simulink library "PczSimLib"  (R2022a)
settings: Solver=VariableStepAuto  StartTime=0.0  StopTime=10.0  RelTol=1e-3
undefined symbols (not defined in the file or in its folder): beta, PczSimLib_R2020b, Reshapers
libraries: dspswit3 x6, simulink x3
(part 2 of 2)

== matlab function PczSimLib/QArm blocks/Torque to pwm (corrected) 2022.04.28./Tau(u,x) ==
  data: params input; u input; x input; Tau output; mL input
function Tau = qarm_Tau(params,u,x,mL)
%#codegen

%    This function was generated by the Symbolic Math Toolbox version 8.7.
%    12-May-2021 15:32:53

%% in1 = u = dd(Theta), in2 = x = [ Theta ; d(Theta) ] , Tau = M(Theta) dd(Theta) + B(Theta) d(Theta) d(Theta) + C(Theta) d(Theta)^2 + G(Theta)
I1A = params(10,:);
I2A = params(11,:);
I3A = params(13,:);
I4A = params(15,:);
I2L = params(12,:);
I3L = params(14,:);
I4L = params(16,:);
payload = mL;
domega1 = u(1,:);
domega2 = u(2,:);
domega3 = u(3,:);
domega4 = u(4,:);
g = params(1,:);
l2 = params(2,:);
l3 = params(3,:);
lc2 = params(4,:);
lc3 = params(5,:);
lc4 = params(6,:);
m2 = params(7,:);
m3 = params(8,:);
m4 = params(9,:);
omega1 = x(5,:);
omega2 = x(6,:);
omega3 = x(7,:);
omega4 = x(8,:);
theta2 = x(2,:);
theta3 = x(3,:);
t2 = cos(theta2);
t3 = cos(theta3);
t4 = sin(theta2);
t5 = sin(theta3);
t6 = theta2+theta3;
t7 = l2.^2;
t8 = l3.^2;
t9 = lc3.^2;
t10 = omega1.^2;
t16 = -l3;
t17 = -lc2;
t18 = -lc4;
t11 = t2.^2;
t12 = l2.*t2;
t13 = cos(t6);
t14 = l2.*t5;
t15 = sin(t6);
t20 = m3.*t9;
t21 = payload.*t8;
t24 = l2.*lc3.*m3.*t3;
t25 = l2.*l3.*payload.*t3;
t27 = l2+t17;
t28 = l3+t18;
t19 = l3.*t14;
t22 = t13.^2;
t23 = t15.^2;
t26 = lc3.*m3.*t14;
t29 = -t12;
t30 = t14.*t16;
t31 = I4A.*omega1.*omega4.*t15;
t33 = t27.^2;
t34 = t28.^2;
t35 = I3A.*t13.*t15;
t36 = I4A.*t13.*t15;
t37 = I3L.*t13.*t15;
t38 = I4L.*t13.*t15;
t39 = lc3.*m3.*t12.*t13;
t40 = l3.*payload.*t12.*t13;
t42 = lc4+t14+t16;
t54 = t13.*t15.*t21;
t56 = t13.*t15.*t20;
t62 = m4.*t12.*t13.*t28;
t32 = -t26;
t41 = -t31;
t43 = t35.*2.0;
t44 = t36.*2.0;
t45 = t37.*2.0;
t46 = t38.*2.0;
t47 = t39.*2.0;
t48 = t40.*2.0;
t49 = t8+t30;
t50 = -t37;
t52 = -t38;
t57 = t54.*2.0;
t58 = t56.*2.0;
t59 = -t54;
t63 = -t56;
t65 = t62.*2.0;
t66 = m4.*t13.*t15.*t34;
t67 = m4.*t28.*t42;
t51 = -t45;
t53 = -t46;
t55 = payload.*t49;
t60 = -t57;
t64 = -t58;
t68 = t66.*2.0;
t69 = -t66;
t71 = -t67;
t61 = -t55;
t70 = -t68;
t72 = I3L+I4L+t20+t32+t61+t71;
mt1 = [domega1.*(I1A+I3A.*t22+I4A.*t22+I2L.*t11+I3L.*t23+I4L.*t23+t20.*t23+t21.*t23+I2A.*t4.^2+m3.*t7.*t11+m4.*t7.*t11+m2.*t11.*t33+m4.*t23.*t34+payload.*t7.*t11-lc3.*m3.*t12.*t15.*2.0-l3.*payload.*t12.*t15.*2.0-m4.*t12.*t15.*t28.*2.0)-omega1.*omega3.*(t43+t44+t47+t48+t51+t53+t60+t64+t65+t70)-I4A.*domega4.*t13-omega1.*omega2.*(t43+t44+t47+t48+t51+t53+t60+t64+t65+t70-I2A.*t2.*t4.*2.0+I2L.*t2.*t4.*2.0+m3.*t2.*t4.*t7.*2.0+m4.*t2.*t4.*t7.*2.0+m2.*t2.*t4.*t33.*2.0+payload.*t2.*t4.*t7.*2.0-l2.*lc3.*m3.*t4.*t15.*2.0-l2.*l3.*payload.*t4.*t15.*2.0-l2.*m4.*t4.*t15.*t28.*2.0)+I4A.*omega2.*omega4.*t15+I4A.*omega3.*omega4.*t15];
mt2 = [t41+domega2.*(I2L+I3L+I4L+t20+t21-t26.*2.0+m3.*t7+m2.*t33+payload.*t7-payload.*t19.*2.0+m4.*(l2+t28).^2)+domega3.*t72+t10.*(t35+t36+t39+t40+t50+t52+t59+t62+t63+t69-I2A.*t2.*t4+I2L.*t2.*t4+m3.*t2.*t4.*t7+m4.*t2.*t4.*t7+m2.*t2.*t4.*t33+payload.*t2.*t4.*t7-l2.*lc3.*m3.*t4.*t15-l2.*m4.*t4.*t15.*t28+l2.*payload.*t4.*t15.*t16)-omega3.^2.*(t24+l2.*m4.*t3.*t28+l2.*payload.*t3.*t16)-g.*(m3.*(t12-lc3.*t15)+m4.*(t12-t15.*t28)+payload.*(t12+t15.*t16)+m2.*t2.*t27)-omega2.*omega3.*(t24.*2.0+t25.*2.0)];
mt3 = [t41+g.*(lc3.*m3.*t15+l3.*payload.*t15+m4.*t15.*t28)+domega2.*t72+omega2.^2.*(t24+t25)+t10.*(t35+t36+t39+t40+t50+t52+t59+t62+t63+t69)+domega3.*(I3L+I4L+t20+t21+m4.*t34),I4A.*domega4-I4A.*domega1.*t13+I4A.*omega1.*omega2.*t15+I4A.*omega1.*omega3.*t15];
Tau = reshape([mt1,mt2,mt3],4,1);

== matlab function PczSimLib/QArm blocks/Torque to pwm (corrected) 2022.05.20./Tau(u,x) ==
  data: params input; u input; x input; Tau output; mL input
function Tau = qarm_Tau(params,u,x,mL)
%#codegen

%    This function was generated by the Symbolic Math Toolbox version 8.7.
%    12-May-2021 15:32:53

%% in1 = u = dd(Theta), in2 = x = [ Theta ; d(Theta) ] , Tau = M(Theta) dd(Theta) + B(Theta) d(Theta) d(Theta) + C(Theta) d(Theta)^2 + G(Theta)
I1A = params(10,:);
I2A = params(11,:);
I3A = params(13,:);
I4A = params(15,:);
I2L = params(12,:);
I3L = params(14,:);
I4L = params(16,:);
payload = mL;
domega1 = u(1,:);
domega2 = u(2,:);
domega3 = u(3,:);
domega4 = u(4,:);
g = params(1,:);
l2 = params(2,:);
l3 = params(3,:);
lc2 = params(4,:);
lc3 = params(5,:);
lc4 = params(6,:);
m2 = params(7,:);
m3 = params(8,:);
m4 = params(9,:);
omega1 = x(5,:);
omega2 = x(6,:);
omega3 = x(7,:);
omega4 = x(8,:);
theta2 = x(2,:);
theta3 = x(3,:);
t2 = cos(theta2);
t3 = cos(theta3);
t4 = sin(theta2);
t5 = sin(theta3);
t6 = theta2+theta3;
t7 = l2.^2;
t8 = l3.^2;
t9 = lc3.^2;
t10 = omega1.^2;
t16 = -l3;
t17 = -lc2;
t18 = -lc4;
t11 = t2.^2;
t12 = l2.*t2;
t13 = cos(t6);
t14 = l2.*t5;
t15 = sin(t6);
t20 = m3.*t9;
t21 = payload.*t8;
t24 = l2.*lc3.*m3.*t3;
t25 = l2.*l3.*payload.*t3;
t27 = l2+t17;
t28 = l3+t18;
t19 = l3.*t14;
t22 = t13.^2;
t23 = t15.^2;
t26 = lc3.*m3.*t14;
t29 = -t12;
t30 = t14.*t16;
t31 = I4A.*omega1.*omega4.*t15;
t33 = t27.^2;
t34 = t28.^2;
t35 = I3A.*t13.*t15;
t36 = I4A.*t13.*t15;
t37 = I3L.*t13.*t15;
t38 = I4L.*t13.*t15;
t39 = lc3.*m3.*t12.*t13;
t40 = l3.*payload.*t12.*t13;
t42 = lc4+t14+t16;
t54 = t13.*t15.*t21;
t56 = t13.*t15.*t20;
t62 = m4.*t12.*t13.*t28;
t32 = -t26;
t41 = -t31;
t43 = t35.*2.0;
t44 = t36.*2.0;
t45 = t37.*2.0;
t46 = t38.*2.0;
t47 = t39.*2.0;
t48 = t40.*2.0;
t49 = t8+t30;
t50 = -t37;
t52 = -t38;
t57 = t54.*2.0;
t58 = t56.*2.0;
t59 = -t54;
t63 = -t56;
t65 = t62.*2.0;
t66 = m4.*t13.*t15.*t34;
t67 = m4.*t28.*t42;
t51 = -t45;
t53 = -t46;
t55 = payload.*t49;
t60 = -t57;
t64 = -t58;
t68 = t66.*2.0;
t69 = -t66;
t71 = -t67;
t61 = -t55;
t70 = -t68;
t72 = I3L+I4L+t20+t32+t61+t71;
mt1 = [domega1.*(I1A+I3A.*t22+I4A.*t22+I2L.*t11+I3L.*t23+I4L.*t23+t20.*t23+t21.*t23+I2A.*t4.^2+m3.*t7.*t11+m4.*t7.*t11+m2.*t11.*t33+m4.*t23.*t34+payload.*t7.*t11-lc3.*m3.*t12.*t15.*2.0-l3.*payload.*t12.*t15.*2.0-m4.*t12.*t15.*t28.*2.0)-omega1.*omega3.*(t43+t44+t47+t48+t51+t53+t60+t64+t65+t70)-I4A.*domega4.*t13-omega1.*omega2.*(t43+t44+t47+t48+t51+t53+t60+t64+t65+t70-I2A.*t2.*t4.*2.0+I2L.*t2.*t4.*2.0+m3.*t2.*t4.*t7.*2.0+m4.*t2.*t4.*t7.*2.0+m2.*t2.*t4.*t33.*2.0+payload.*t2.*t4.*t7.*2.0-l2.*lc3.*m3.*t4.*t15.*2.0-l2.*l3.*payload.*t4.*t15.*2.0-l2.*m4.*t4.*t15.*t28.*2.0)+I4A.*omega2.*omega4.*t15+I4A.*omega3.*omega4.*t15];
mt2 = [t41+domega2.*(I2L+I3L+I4L+t20+t21-t26.*2.0+m3.*t7+m2.*t33+payload.*t7-payload.*t19.*2.0+m4.*(l2+t28).^2)+domega3.*t72+t10.*(t35+t36+t39+t40+t50+t52+t59+t62+t63+t69-I2A.*t2.*t4+I2L.*t2.*t4+m3.*t2.*t4.*t7+m4.*t2.*t4.*t7+m2.*t2.*t4.*t33+payload.*t2.*t4.*t7-l2.*lc3.*m3.*t4.*t15-l2.*m4.*t4.*t15.*t28+l2.*payload.*t4.*t15.*t16)-omega3.^2.*(t24+l2.*m4.*t3.*t28+l2.*payload.*t3.*t16)-g.*(m3.*(t12-lc3.*t15)+m4.*(t12-t15.*t28)+payload.*(t12+t15.*t16)+m2.*t2.*t27)-omega2.*omega3.*(t24.*2.0+t25.*2.0)];
mt3 = [t41+g.*(lc3.*m3.*t15+l3.*payload.*t15+m4.*t15.*t28)+domega2.*t72+omega2.^2.*(t24+t25)+t10.*(t35+t36+t39+t40+t50+t52+t59+t62+t63+t69)+domega3.*(I3L+I4L+t20+t21+m4.*t34),I4A.*domega4-I4A.*domega1.*t13+I4A.*omega1.*omega2.*t15+I4A.*omega1.*omega3.*t15];
Tau = reshape([mt1,mt2,mt3],4,1);

== matlab function PczSimLib/QArm blocks/Torque to pwm DEPRECATED/Tau(u,x) ==
  data: params input; u input; x input; Tau output; mL input
function Tau = qarm_Tau(params,u,x,mL)
%#codegen

%    This function was generated by the Symbolic Math Toolbox version 8.7.
%    12-May-2021 15:32:53

%% in1 = u = dd(Theta), in2 = x = [ Theta ; d(Theta) ] , Tau = M(Theta) dd(Theta) + B(Theta) d(Theta) d(Theta) + C(Theta) d(Theta)^2 + G(Theta)
I1A = params(10,:);
I2A = params(11,:);
I3A = params(13,:);
I4A = params(15,:);
I2L = params(12,:);
I3L = params(14,:);
I4L = params(16,:);
payload = mL;
domega1 = u(1,:);
domega2 = u(2,:);
domega3 = u(3,:);
domega4 = u(4,:);
g = params(1,:);
l2 = params(2,:);
l3 = params(3,:);
lc2 = params(4,:);
lc3 = params(5,:);
lc4 = params(6,:);
m2 = params(7,:);
m3 = params(8,:);
m4 = params(9,:);
omega1 = x(5,:);
omega2 = x(6,:);
omega3 = x(7,:);
omega4 = x(8,:);
theta2 = x(2,:);
theta3 = x(3,:);
t2 = cos(theta2);
t3 = cos(theta3);
t4 = sin(theta2);
t5 = sin(theta3);
t6 = theta2+theta3;
t7 = l2.^2;
t8 = l3.^2;
t9 = lc3.^2;
t10 = omega1.^2;
t16 = -l3;
t17 = -lc2;
t18 = -lc4;
t11 = t2.^2;
t12 = l2.*t2;
t13 = cos(t6);
t14 = l2.*t5;
t15 = sin(t6);
t20 = m3.*t9;
t21 = payload.*t8;
t24 = l2.*lc3.*m3.*t3;
t25 = l2.*l3.*payload.*t3;
t27 = l2+t17;
t28 = l3+t18;
t19 = l3.*t14;
t22 = t13.^2;
t23 = t15.^2;
t26 = lc3.*m3.*t14;
t29 = -t12;
t30 = t14.*t16;
t31 = I4A.*omega1.*omega4.*t15;
t33 = t27.^2;
t34 = t28.^2;
t35 = I3A.*t13.*t15;
t36 = I4A.*t13.*t15;
t37 = I3L.*t13.*t15;
t38 = I4L.*t13.*t15;
t39 = lc3.*m3.*t12.*t13;
t40 = l3.*payload.*t12.*t13;
t42 = lc4+t14+t16;
t54 = t13.*t15.*t21;
t56 = t13.*t15.*t20;
t62 = m4.*t12.*t13.*t28;
t32 = -t26;
t41 = -t31;
t43 = t35.*2.0;
t44 = t36.*2.0;
t45 = t37.*2.0;
t46 = t38.*2.0;
t47 = t39.*2.0;
t48 = t40.*2.0;
t49 = t8+t30;
t50 = -t37;
t52 = -t38;
t57 = t54.*2.0;
t58 = t56.*2.0;
t59 = -t54;
t63 = -t56;
t65 = t62.*2.0;
t66 = m4.*t13.*t15.*t34;
t67 = m4.*t28.*t42;
t51 = -t45;
t53 = -t46;
t55 = payload.*t49;
t60 = -t57;
t64 = -t58;
t68 = t66.*2.0;
t69 = -t66;
t71 = -t67;
t61 = -t55;
t70 = -t68;
t72 = I3L+I4L+t20+t32+t61+t71;
mt1 = [domega1.*(I1A+I3A.*t22+I4A.*t22+I2L.*t11+I3L.*t23+I4L.*t23+t20.*t23+t21.*t23+I2A.*t4.^2+m3.*t7.*t11+m4.*t7.*t11+m2.*t11.*t33+m4.*t23.*t34+payload.*t7.*t11-lc3.*m3.*t12.*t15.*2.0-l3.*payload.*t12.*t15.*2.0-m4.*t12.*t15.*t28.*2.0)-omega1.*omega3.*(t43+t44+t47+t48+t51+t53+t60+t64+t65+t70)-I4A.*domega4.*t13-omega1.*omega2.*(t43+t44+t47+t48+t51+t53+t60+t64+t65+t70-I2A.*t2.*t4.*2.0+I2L.*t2.*t4.*2.0+m3.*t2.*t4.*t7.*2.0+m4.*t2.*t4.*t7.*2.0+m2.*t2.*t4.*t33.*2.0+payload.*t2.*t4.*t7.*2.0-l2.*lc3.*m3.*t4.*t15.*2.0-l2.*l3.*payload.*t4.*t15.*2.0-l2.*m4.*t4.*t15.*t28.*2.0)+I4A.*omega2.*omega4.*t15+I4A.*omega3.*omega4.*t15];
mt2 = [t41+domega2.*(I2L+I3L+I4L+t20+t21-t26.*2.0+m3.*t7+m2.*t33+payload.*t7-payload.*t19.*2.0+m4.*(l2+t28).^2)+domega3.*t72+t10.*(t35+t36+t39+t40+t50+t52+t59+t62+t63+t69-I2A.*t2.*t4+I2L.*t2.*t4+m3.*t2.*t4.*t7+m4.*t2.*t4.*t7+m2.*t2.*t4.*t33+payload.*t2.*t4.*t7-l2.*lc3.*m3.*t4.*t15-l2.*m4.*t4.*t15.*t28+l2.*payload.*t4.*t15.*t16)-omega3.^2.*(t24+l2.*m4.*t3.*t28+l2.*payload.*t3.*t16)-g.*(m3.*(t12-lc3.*t15)+m4.*(t12-t15.*t28)+payload.*(t12+t15.*t16)+m2.*t2.*t27)-omega2.*omega3.*(t24.*2.0+t25.*2.0)];
mt3 = [t41+g.*(lc3.*m3.*t15+l3.*payload.*t15+m4.*t15.*t28)+domega2.*t72+omega2.^2.*(t24+t25)+t10.*(t35+t36+t39+t40+t50+t52+t59+t62+t63+t69)+domega3.*(I3L+I4L+t20+t21+m4.*t34),I4A.*domega4-I4A.*domega1.*t13+I4A.*omega1.*omega2.*t15+I4A.*omega1.*omega3.*t15];
Tau = reshape([mt1,mt2,mt3],4,1);
